simulink model "simple_streaming_txrx"  (Simulink 6.6)
settings: Solver=ode45  StartTime=0.0  StopTime=inf  RelTol=1e-3
InitFcn:
  | simple_streaming_init
StartFcn:
  | simple_streaming_init
undefined symbols (not defined in the file): dmf, gcbh, get, modConstellation_qam16, modConstellation_qam64, modConstellation_qpsk, rcosfir, symbolRomLen, txLSFR_initValues, txLSFR_polynomials, viqAvgLen, xlBlockLoadCallback, xlGetSimulinkPeriod
libraries: xbsIndex_r4 x506, commchan3 x2, commsink2 x1
(part 2 of 5)

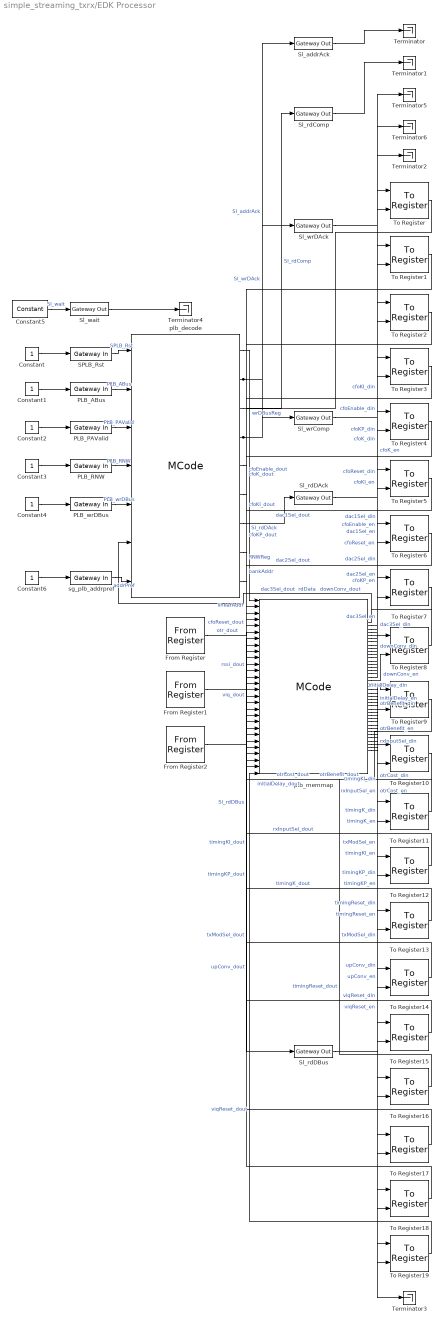
== system simple_streaming_txrx/EDK Processor ==
  Constant{,1..4,6} (6 alike) : Constant
  Constant5 : xbsIndex_r4/Constant  arith_type=Unsigned  const=0  n_bits=1  bin_pt=0  explicit_period=on  period=xlGetSimulinkPeriod(gcb)  equ=P=C  opselect=C  inp2=PCIN>>17  opr=+  inp1=P  carry=CIN  dbl_ovrd=off  block_type=constant
      settings: block_version=10.1.2
  From Register : xbsIndex_r4/From Register  shared_memory_name='otr'  init=0  period=xlGetSimulinkPeriod(gcb)  ownership=Owned and initialized elsewhere  arith_type=Unsigned  n_bits=32  bin_pt=0  dbl_ovrd=off  block_type=fromreg
      settings: AttributesFormatString=<< %<shared_memory_name> >>  infoedit="Register block that reads data to a shared memory register.  Delay of one sample period."  block_version=10.1.2
  From Register1 : xbsIndex_r4/From Register  shared_memory_name='rssi'  init=0  period=xlGetSimulinkPeriod(gcb)  ownership=Owned and initialized elsewhere  arith_type=Unsigned  n_bits=32  bin_pt=0  dbl_ovrd=off  block_type=fromreg
      settings: AttributesFormatString=<< %<shared_memory_name> >>  infoedit="Register block that reads data to a shared memory register.  Delay of one sample period."  block_version=10.1.2
  From Register2 : xbsIndex_r4/From Register  shared_memory_name='viq'  init=0  period=xlGetSimulinkPeriod(gcb)  ownership=Owned and initialized elsewhere  arith_type=Unsigned  n_bits=32  bin_pt=0  dbl_ovrd=off  block_type=fromreg
      settings: AttributesFormatString=<< %<shared_memory_name> >>  infoedit="Register block that reads data to a shared memory register.  Delay of one sample period."  block_version=10.1.2
  PLB_ABus : xbsIndex_r4/Gateway In  arith_type=Unsigned  n_bits=32  bin_pt=0  quantization="Round  (unbiased: +/- Inf)"  overflow=Saturate  period=xlGetSimulinkPeriod(gcb)  dbl_ovrd=off  timing_constraint=None  locs_specified=off  LOCs={}  block_type=gatewayin
      settings: infoedit="Gateway in block.  Converts inputs of type Simulink integer, double and fixed point to  Xilinx fixed point type.<P><P>Hardware notes:  In hardware these blocks become top level input ports."  sginterface={'Xilinx'=>{'jtaghwcosim'=>{'non_memory_mapped_port'=>'PLB_ABus'}},'iopad'=>{'constraint'=>'#'}}  block_version=10.1.2
  PLB_PAValid : xbsIndex_r4/Gateway In  arith_type=Unsigned  n_bits=1  bin_pt=0  quantization="Round  (unbiased: +/- Inf)"  overflow=Saturate  period=xlGetSimulinkPeriod(gcb)  dbl_ovrd=off  timing_constraint=None  locs_specified=off  LOCs={}  block_type=gatewayin
      settings: infoedit="Gateway in block.  Converts inputs of type Simulink integer, double and fixed point to  Xilinx fixed point type.<P><P>Hardware notes:  In hardware these blocks become top level input ports."  sginterface={'Xilinx'=>{'jtaghwcosim'=>{'non_memory_mapped_port'=>'PLB_PAValid'}},'iopad'=>{'constraint'=>'#'}}  block_version=10.1.2
  PLB_RNW : xbsIndex_r4/Gateway In  arith_type=Unsigned  n_bits=1  bin_pt=0  quantization="Round  (unbiased: +/- Inf)"  overflow=Saturate  period=xlGetSimulinkPeriod(gcb)  dbl_ovrd=off  timing_constraint=None  locs_specified=off  LOCs={}  block_type=gatewayin
      settings: infoedit="Gateway in block.  Converts inputs of type Simulink integer, double and fixed point to  Xilinx fixed point type.<P><P>Hardware notes:  In hardware these blocks become top level input ports."  sginterface={'Xilinx'=>{'jtaghwcosim'=>{'non_memory_mapped_port'=>'PLB_RNW'}},'iopad'=>{'constraint'=>'#'}}  block_version=10.1.2
  PLB_wrDBus : xbsIndex_r4/Gateway In  arith_type=Unsigned  n_bits=32  bin_pt=0  quantization="Round  (unbiased: +/- Inf)"  overflow=Saturate  period=xlGetSimulinkPeriod(gcb)  dbl_ovrd=off  timing_constraint=None  locs_specified=off  LOCs={}  block_type=gatewayin
      settings: infoedit="Gateway in block.  Converts inputs of type Simulink integer, double and fixed point to  Xilinx fixed point type.<P><P>Hardware notes:  In hardware these blocks become top level input ports."  sginterface={'Xilinx'=>{'jtaghwcosim'=>{'non_memory_mapped_port'=>'PLB_wrDBus'}},'iopad'=>{'constraint'=>'#'}}  block_version=10.1.2
  SPLB_Rst : xbsIndex_r4/Gateway In  arith_type=Unsigned  n_bits=1  bin_pt=0  quantization="Round  (unbiased: +/- Inf)"  overflow=Saturate  period=xlGetSimulinkPeriod(gcb)  dbl_ovrd=off  timing_constraint=None  locs_specified=off  LOCs={}  block_type=gatewayin
      settings: infoedit="Gateway in block.  Converts inputs of type Simulink integer, double and fixed point to  Xilinx fixed point type.<P><P>Hardware notes:  In hardware these blocks become top level input ports."  sginterface={'Xilinx'=>{'jtaghwcosim'=>{'non_memory_mapped_port'=>'SPLB_Rst'}},'iopad'=>{'constraint'=>'#'}}  block_version=10.1.2
  Sl_addrAck : xbsIndex_r4/Gateway Out  hdl_port=on  timing_constraint=None  locs_specified=off  LOCs={}  block_type=gatewayout
      settings: infoedit="Gateway out block.  Converts Xilinx fixed point inputs into ouputs of type Simulink integer, double, or fixed point.<P><P>Hardware notes:  In hardware these blocks become top level output ports or are discarded, depending on how they are configured."  sginterface={'Xilinx'=>{'jtaghwcosim'=>{'non_memory_mapped_port'=>'Sl_addrAck'}},'iopad'=>{'constraint'=>'#'}}  block_version=10.1.2
  Sl_rdComp : xbsIndex_r4/Gateway Out  hdl_port=on  timing_constraint=None  locs_specified=off  LOCs={}  block_type=gatewayout
      settings: infoedit="Gateway out block.  Converts Xilinx fixed point inputs into ouputs of type Simulink integer, double, or fixed point.<P><P>Hardware notes:  In hardware these blocks become top level output ports or are discarded, depending on how they are configured."  sginterface={'Xilinx'=>{'jtaghwcosim'=>{'non_memory_mapped_port'=>'Sl_rdComp'}},'iopad'=>{'constraint'=>'#'}}  block_version=10.1.2
  Sl_rdDAck : xbsIndex_r4/Gateway Out  hdl_port=on  timing_constraint=None  locs_specified=off  LOCs={}  block_type=gatewayout
      settings: infoedit="Gateway out block.  Converts Xilinx fixed point inputs into ouputs of type Simulink integer, double, or fixed point.<P><P>Hardware notes:  In hardware these blocks become top level output ports or are discarded, depending on how they are configured."  sginterface={'Xilinx'=>{'jtaghwcosim'=>{'non_memory_mapped_port'=>'Sl_rdDAck'}},'iopad'=>{'constraint'=>'#'}}  block_version=10.1.2
  Sl_rdDBus : xbsIndex_r4/Gateway Out  hdl_port=on  timing_constraint=None  locs_specified=off  LOCs={}  block_type=gatewayout
      settings: infoedit="Gateway out block.  Converts Xilinx fixed point inputs into ouputs of type Simulink integer, double, or fixed point.<P><P>Hardware notes:  In hardware these blocks become top level output ports or are discarded, depending on how they are configured."  sginterface={'Xilinx'=>{'jtaghwcosim'=>{'non_memory_mapped_port'=>'Sl_rdDBus'}},'iopad'=>{'constraint'=>'#'}}  block_version=10.1.2
  Sl_wait : xbsIndex_r4/Gateway Out  hdl_port=on  timing_constraint=None  locs_specified=off  LOCs={}  block_type=gatewayout
      settings: infoedit="Gateway out block.  Converts Xilinx fixed point inputs into ouputs of type Simulink integer, double, or fixed point.<P><P>Hardware notes:  In hardware these blocks become top level output ports or are discarded, depending on how they are configured."  sginterface={'Xilinx'=>{'jtaghwcosim'=>{'non_memory_mapped_port'=>'Sl_wait'}},'iopad'=>{'constraint'=>'#'}}  block_version=10.1.2
  Sl_wrComp : xbsIndex_r4/Gateway Out  hdl_port=on  timing_constraint=None  locs_specified=off  LOCs={}  block_type=gatewayout
      settings: infoedit="Gateway out block.  Converts Xilinx fixed point inputs into ouputs of type Simulink integer, double, or fixed point.<P><P>Hardware notes:  In hardware these blocks become top level output ports or are discarded, depending on how they are configured."  sginterface={'Xilinx'=>{'jtaghwcosim'=>{'non_memory_mapped_port'=>'Sl_wrComp'}},'iopad'=>{'constraint'=>'#'}}  block_version=10.1.2
  Sl_wrDAck : xbsIndex_r4/Gateway Out  hdl_port=on  timing_constraint=None  locs_specified=off  LOCs={}  block_type=gatewayout
      settings: infoedit="Gateway out block.  Converts Xilinx fixed point inputs into ouputs of type Simulink integer, double, or fixed point.<P><P>Hardware notes:  In hardware these blocks become top level output ports or are discarded, depending on how they are configured."  sginterface={'Xilinx'=>{'jtaghwcosim'=>{'non_memory_mapped_port'=>'Sl_wrDAck'}},'iopad'=>{'constraint'=>'#'}}  block_version=10.1.2
  Terminator{,1..6} (7 alike) : Terminator
  To Register : xbsIndex_r4/To Register  shared_memory_name='cfoEnable'  init=0  ownership=Owned and initialized elsewhere  explicit_data_type=on  arith_type=Unsigned  n_bits=1  bin_pt=0  dbl_ovrd=off  block_type=toreg
      settings: AttributesFormatString=<< %<shared_memory_name> >>  infoedit="Register block that writes data to a shared memory register.  Delay of one sample period."  block_version=10.1.2
  To Register1 : xbsIndex_r4/To Register  shared_memory_name='cfoK'  init=0  ownership=Owned and initialized elsewhere  explicit_data_type=on  arith_type=Unsigned  n_bits=32  bin_pt=0  dbl_ovrd=off  block_type=toreg
      settings: AttributesFormatString=<< %<shared_memory_name> >>  infoedit="Register block that writes data to a shared memory register.  Delay of one sample period."  block_version=10.1.2
  To Register10 : xbsIndex_r4/To Register  shared_memory_name='otrBenefit'  init=0  ownership=Owned and initialized elsewhere  explicit_data_type=on  arith_type=Unsigned  n_bits=32  bin_pt=0  dbl_ovrd=off  block_type=toreg
      settings: AttributesFormatString=<< %<shared_memory_name> >>  infoedit="Register block that writes data to a shared memory register.  Delay of one sample period."  block_version=10.1.2
  To Register11 : xbsIndex_r4/To Register  shared_memory_name='otrCost'  init=0  ownership=Owned and initialized elsewhere  explicit_data_type=on  arith_type=Unsigned  n_bits=32  bin_pt=0  dbl_ovrd=off  block_type=toreg
      settings: AttributesFormatString=<< %<shared_memory_name> >>  infoedit="Register block that writes data to a shared memory register.  Delay of one sample period."  block_version=10.1.2
  To Register12 : xbsIndex_r4/To Register  shared_memory_name='rxInputSel'  init=0  ownership=Owned and initialized elsewhere  explicit_data_type=on  arith_type=Unsigned  n_bits=2  bin_pt=0  dbl_ovrd=off  block_type=toreg
      settings: AttributesFormatString=<< %<shared_memory_name> >>  infoedit="Register block that writes data to a shared memory register.  Delay of one sample period."  block_version=10.1.2
  To Register13 : xbsIndex_r4/To Register  shared_memory_name='timingK'  init=0  ownership=Owned and initialized elsewhere  explicit_data_type=on  arith_type=Unsigned  n_bits=32  bin_pt=0  dbl_ovrd=off  block_type=toreg
      settings: AttributesFormatString=<< %<shared_memory_name> >>  infoedit="Register block that writes data to a shared memory register.  Delay of one sample period."  block_version=10.1.2
  To Register14 : xbsIndex_r4/To Register  shared_memory_name='timingKI'  init=0  ownership=Owned and initialized elsewhere  explicit_data_type=on  arith_type=Unsigned  n_bits=32  bin_pt=0  dbl_ovrd=off  block_type=toreg
      settings: AttributesFormatString=<< %<shared_memory_name> >>  infoedit="Register block that writes data to a shared memory register.  Delay of one sample period."  block_version=10.1.2
  To Register15 : xbsIndex_r4/To Register  shared_memory_name='timingKP'  init=0  ownership=Owned and initialized elsewhere  explicit_data_type=on  arith_type=Unsigned  n_bits=32  bin_pt=0  dbl_ovrd=off  block_type=toreg
      settings: AttributesFormatString=<< %<shared_memory_name> >>  infoedit="Register block that writes data to a shared memory register.  Delay of one sample period."  block_version=10.1.2
  To Register16 : xbsIndex_r4/To Register  shared_memory_name='timingReset'  init=0  ownership=Owned and initialized elsewhere  explicit_data_type=on  arith_type=Unsigned  n_bits=1  bin_pt=0  dbl_ovrd=off  block_type=toreg
      settings: AttributesFormatString=<< %<shared_memory_name> >>  infoedit="Register block that writes data to a shared memory register.  Delay of one sample period."  block_version=10.1.2
  To Register17 : xbsIndex_r4/To Register  shared_memory_name='txModSel'  init=0  ownership=Owned and initialized elsewhere  explicit_data_type=on  arith_type=Unsigned  n_bits=2  bin_pt=0  dbl_ovrd=off  block_type=toreg
      settings: AttributesFormatString=<< %<shared_memory_name> >>  infoedit="Register block that writes data to a shared memory register.  Delay of one sample period."  block_version=10.1.2
  To Register18 : xbsIndex_r4/To Register  shared_memory_name='upConv'  init=0  ownership=Owned and initialized elsewhere  explicit_data_type=on  arith_type=Unsigned  n_bits=32  bin_pt=0  dbl_ovrd=off  block_type=toreg
      settings: AttributesFormatString=<< %<shared_memory_name> >>  infoedit="Register block that writes data to a shared memory register.  Delay of one sample period."  block_version=10.1.2
  To Register19 : xbsIndex_r4/To Register  shared_memory_name='viqReset'  init=0  ownership=Owned and initialized elsewhere  explicit_data_type=on  arith_type=Unsigned  n_bits=1  bin_pt=0  dbl_ovrd=off  block_type=toreg
      settings: AttributesFormatString=<< %<shared_memory_name> >>  infoedit="Register block that writes data to a shared memory register.  Delay of one sample period."  block_version=10.1.2
  To Register2 : xbsIndex_r4/To Register  shared_memory_name='cfoKI'  init=0  ownership=Owned and initialized elsewhere  explicit_data_type=on  arith_type=Unsigned  n_bits=32  bin_pt=0  dbl_ovrd=off  block_type=toreg
      settings: AttributesFormatString=<< %<shared_memory_name> >>  infoedit="Register block that writes data to a shared memory register.  Delay of one sample period."  block_version=10.1.2
  To Register3 : xbsIndex_r4/To Register  shared_memory_name='cfoKP'  init=0  ownership=Owned and initialized elsewhere  explicit_data_type=on  arith_type=Unsigned  n_bits=32  bin_pt=0  dbl_ovrd=off  block_type=toreg
      settings: AttributesFormatString=<< %<shared_memory_name> >>  infoedit="Register block that writes data to a shared memory register.  Delay of one sample period."  block_version=10.1.2
  To Register4 : xbsIndex_r4/To Register  shared_memory_name='cfoReset'  init=0  ownership=Owned and initialized elsewhere  explicit_data_type=on  arith_type=Unsigned  n_bits=1  bin_pt=0  dbl_ovrd=off  block_type=toreg
      settings: AttributesFormatString=<< %<shared_memory_name> >>  infoedit="Register block that writes data to a shared memory register.  Delay of one sample period."  block_version=10.1.2
  To Register5 : xbsIndex_r4/To Register  shared_memory_name='dac1Sel'  init=0  ownership=Owned and initialized elsewhere  explicit_data_type=on  arith_type=Unsigned  n_bits=2  bin_pt=0  dbl_ovrd=off  block_type=toreg
      settings: AttributesFormatString=<< %<shared_memory_name> >>  infoedit="Register block that writes data to a shared memory register.  Delay of one sample period."  block_version=10.1.2
  To Register6 : xbsIndex_r4/To Register  shared_memory_name='dac2Sel'  init=0  ownership=Owned and initialized elsewhere  explicit_data_type=on  arith_type=Unsigned  n_bits=2  bin_pt=0  dbl_ovrd=off  block_type=toreg
      settings: AttributesFormatString=<< %<shared_memory_name> >>  infoedit="Register block that writes data to a shared memory register.  Delay of one sample period."  block_version=10.1.2
  To Register7 : xbsIndex_r4/To Register  shared_memory_name='dac3Sel'  init=0  ownership=Owned and initialized elsewhere  explicit_data_type=on  arith_type=Unsigned  n_bits=1  bin_pt=0  dbl_ovrd=off  block_type=toreg
      settings: AttributesFormatString=<< %<shared_memory_name> >>  infoedit="Register block that writes data to a shared memory register.  Delay of one sample period."  block_version=10.1.2
  To Register8 : xbsIndex_r4/To Register  shared_memory_name='downConv'  init=0  ownership=Owned and initialized elsewhere  explicit_data_type=on  arith_type=Unsigned  n_bits=32  bin_pt=0  dbl_ovrd=off  block_type=toreg
      settings: AttributesFormatString=<< %<shared_memory_name> >>  infoedit="Register block that writes data to a shared memory register.  Delay of one sample period."  block_version=10.1.2
  To Register9 : xbsIndex_r4/To Register  shared_memory_name='initialDelay'  init=0  ownership=Owned and initialized elsewhere  explicit_data_type=on  arith_type=Unsigned  n_bits=2  bin_pt=0  dbl_ovrd=off  block_type=toreg
      settings: AttributesFormatString=<< %<shared_memory_name> >>  infoedit="Register block that writes data to a shared memory register.  Delay of one sample period."  block_version=10.1.2
  plb_decode : xbsIndex_r4/MCode  mfname=xlmax  explicit_period=off  period=1  dbl_ovrd=off  enable_stdout=off  enable_debug=off  mfilecontent=|  suppress_output=1  defparams={}  hide_port_list={}  block_type=mcode
      | function [wrDBusReg, addrAck, rdComp, wrDAck, bankAddr, RNWReg, rdDAck, rdDBus, linearAddr] = ...
      |     plb_bus_decode(plbRst, plbABus, plbPAValid, plbRNW, plbWrDBus, rdData, addrPref)
      | 
      | % constant variables (TODO: should pass from outside)
      | ADDRPREF_LEN = 20;
      | BANKADDR_LEN = 2;
      | LINEARADDR_LEN = 8;
      | ABUS_LEN = 32;
      | DBUS_LEN = 32;
      | 
      | % declare and initialize persistent variables
      | % register input bus signals
      | persistent plbRstReg_, plbRstReg_ = xl_state(0, {xlBoolean});
      | persistent plbABusReg_, plbABusReg_ = xl_state(0, {xlUnsigned, ABUS_LEN, 0});
      | persistent plbPAValidReg_, plbPAValidReg_ = xl_state(0, {xlBoolean});
      | persistent plbRNWReg_, plbRNWReg_ = xl_state(0, {xlUnsigned, 1, 0});
      | persistent plbWrDBusReg_, plbWrDBusReg_ = xl_state(0, {xlUnsigned, DBUS_LEN, 0});
      | 
      | % ===== rest of the outputs =====
      | 
      | bankAddr   = xl_slice(plbABusReg_, 2+BANKADDR_LEN+LINEARADDR_LEN-1, 2+LINEARADDR_LEN);
      | linearAddr = xl_slice(plbABusReg_, 2+LINEARADDR_LEN-1, 2);
      | RNWReg = plbRNWReg_;
      | wrDBusReg = plbWrDBusReg_;
      | 
      | % ===== p_select =====
      | 
      | % register PAValid
      | persistent aValidReg, aValidReg = xl_state(0, {xlBoolean});
      | aValidReg = plbPAValidReg_;
      | 
      | % extract and register the address prefix
      | addrPref_in = xl_slice(plbABusReg_, xl_nbits(plbABusReg_)-1, xl_nbits(plbABusReg_)-ADDRPREF_LEN);
      | if addrPref_in == addrPref
      |     ps1 = true;
      | else 
      |     ps1 = false;
      | end 
      | 
      | persistent ps1Reg, ps1Reg = xl_state(0, ps1);
      | ps1Reg = ps1;
      | 
      | ps = xl_and(ps1Reg, aValidReg);
      | 
      | % ===== addrAck =====
      | 
      | % register ps
      | persistent psReg, psReg = xl_state(0, ps);
      | 
      | addrAck = xfix({xlUnsigned, 1, 0}, xl_and(xl_not(plbRstReg_), ps, xl_not(psReg)));
      | 
      | psReg = ps;
      | 
      | % ===== rdComp, rd/wr DAck =====
      |  
      | rdComp1 = xfix({xlUnsigned, 1, 0}, xl_and(addrAck, RNWReg));
      | 
      | NUM_rdCompDelay = 3;
      | persistent rdCompDelay, rdCompDelay = xl_state(zeros(1, NUM_rdCompDelay), rdComp1, NUM_rdCompDelay);
      | rdComp2 = rdCompDelay.back;
      | rdCompDelay.push_front_pop_back(rdComp1);
      | 
      | persistent rdCompReg, rdCompReg = xl_state(0, rdComp1);
      | rdComp = rdCompReg;
      | rdCompReg = rdComp2;
      | 
      | persistent rdDAckReg, rdDAckReg = xl_state(0, rdComp1);
      | rdDAck = rdDAckReg;
      | rdDAckReg = rdComp;
      | 
      | persistent wrDAckReg, wrDAckReg = xl_state(0, addrAck);
      | wrDAck = wrDAckReg;
      | wrDAckReg = xl_and(addrAck, xl_not(RNWReg));
      | 
      | % ===== rdDBus =====
      | 
      | rdSel = xl_or(rdComp2, rdComp);
      | 
      | if rdSel == 1
      |     rdDBus1 = rdData;
      | else
      |     rdDBus1 = 0;
      | end % if
      | 
      | persistent rdDBusReg, rdDBusReg = xl_state(0, rdDBus1);
      | rdDBus = rdDBusReg;
      | rdDBusReg = rdDBus1;
      | 
      | % rdDBus = xl_concat(rdDBus32, rdDBus32);
      | % rdDBus = rdDBus32;
      | 
      | % ===== update the persistent variables =====
      | 
      | plbRstReg_ = plbRst;
      | plbABusReg_ = plbABus;
      | plbPAValidReg_ = plbPAValid;
      | plbRNWReg_ = plbRNW;
      | plbWrDBusReg_ = xl_slice(plbWrDBus, DBUS_LEN-1, 0);
      settings: block_version=10.1.2
  plb_memmap : xbsIndex_r4/MCode  mfname=xlmax  explicit_period=off  period=1  dbl_ovrd=off  enable_stdout=off  enable_debug=off  mfilecontent=|  suppress_output=1  defparams={}  hide_port_list={}  block_type=mcode
      | function [read_bank_out, sm_cfoEnable_din, sm_cfoEnable_en, sm_cfoK_din, sm_cfoK_en, sm_cfoKI_din, sm_cfoKI_en, sm_cfoKP_din, sm_cfoKP_en, sm_cfoReset_din, sm_cfoReset_en, sm_dac1Sel_din, sm_dac1Sel_en, sm_dac2Sel_din, sm_dac2Sel_en, sm_dac3Sel_din, sm_dac3Sel_en, sm_downConv_din, sm_downConv_en, sm_initialDelay_din, sm_initialDelay_en, sm_otrBenefit_din, sm_otrBenefit_en, sm_otrCost_din, sm_otrCost_en, sm_rxInputSel_din, sm_rxInputSel_en, sm_timingK_din, sm_timingK_en, sm_timingKI_din, sm_timingKI_en, sm_timingKP_din, sm_timingKP_en, sm_timingReset_din, sm_timingReset_en, sm_txModSel_din, sm_txModSel_en, sm_upConv_din, sm_upConv_en, sm_viqReset_din, sm_viqReset_en] = plb_memmap_select(wrDBus, bankAddr, linearAddr, RNWReg, addrAck, sm_otr, sm_rssi, sm_viq, sm_cfoEnable, sm_cfoK, sm_cfoKI, sm_cfoKP, sm_cfoReset, sm_dac1Sel, sm_dac2Sel, sm_dac3Sel, sm_downConv, sm_initialDelay, sm_otrBenefit, sm_otrCost, sm_rxInputSel, sm_timingK, sm_timingKI, sm_timingKP, sm_timingReset, sm_txModSel, sm_upConv, sm_viqReset)
      | 
      | 
      | % connvert the input data to UFix_32_0 (the bus data type)
      | % 'From Register' blocks
      | % sm_otr_bus = xfix({xlUnsigned, 32, 0}, 0);
      | sm_otr_bus = xl_force(sm_otr, xlUnsigned, 0);
      | 
      | % sm_rssi_bus = xfix({xlUnsigned, 32, 0}, 0);
      | sm_rssi_bus = xl_force(sm_rssi, xlUnsigned, 0);
      | 
      | % sm_viq_bus = xfix({xlUnsigned, 32, 0}, 0);
      | sm_viq_bus = xl_force(sm_viq, xlUnsigned, 0);
      | 
      | % 'To Register' blocks
      | % sm_cfoEnable_dout = xfix({xlUnsigned, 32, 0}, 0);
      | sm_cfoEnable_dout = xl_force(sm_cfoEnable, xlUnsigned, 0);
      | 
      | % sm_cfoK_dout = xfix({xlUnsigned, 32, 0}, 0);
      | sm_cfoK_dout = xl_force(sm_cfoK, xlUnsigned, 0);
      | 
      | % sm_cfoKI_dout = xfix({xlUnsigned, 32, 0}, 0);
      | sm_cfoKI_dout = xl_force(sm_cfoKI, xlUnsigned, 0);
      | 
      | % sm_cfoKP_dout = xfix({xlUnsigned, 32, 0}, 0);
      | sm_cfoKP_dout = xl_force(sm_cfoKP, xlUnsigned, 0);
      | 
      | % sm_cfoReset_dout = xfix({xlUnsigned, 32, 0}, 0);
      | sm_cfoReset_dout = xl_force(sm_cfoReset, xlUnsigned, 0);
      | 
      | % sm_dac1Sel_dout = xfix({xlUnsigned, 32, 0}, 0);
      | sm_dac1Sel_dout = xl_force(sm_dac1Sel, xlUnsigned, 0);
      | 
      | % sm_dac2Sel_dout = xfix({xlUnsigned, 32, 0}, 0);
      | sm_dac2Sel_dout = xl_force(sm_dac2Sel, xlUnsigned, 0);
      | 
      | % sm_dac3Sel_dout = xfix({xlUnsigned, 32, 0}, 0);
      | sm_dac3Sel_dout = xl_force(sm_dac3Sel, xlUnsigned, 0);
      | 
      | % sm_downConv_dout = xfix({xlUnsigned, 32, 0}, 0);
      | sm_downConv_dout = xl_force(sm_downConv, xlUnsigned, 0);
      | 
      | % sm_initialDelay_dout = xfix({xlUnsigned, 32, 0}, 0);
      | sm_initialDelay_dout = xl_force(sm_initialDelay, xlUnsigned, 0);
      | 
      | % sm_otrBenefit_dout = xfix({xlUnsigned, 32, 0}, 0);
      | sm_otrBenefit_dout = xl_force(sm_otrBenefit, xlUnsigned, 0);
      | 
      | % sm_otrCost_dout = xfix({xlUnsigned, 32, 0}, 0);
      | sm_otrCost_dout = xl_force(sm_otrCost, xlUnsigned, 0);
      | 
      | % sm_rxInputSel_dout = xfix({xlUnsigned, 32, 0}, 0);
      | sm_rxInputSel_dout = xl_force(sm_rxInputSel, xlUnsigned, 0);
      | 
      | % sm_timingK_dout = xfix({xlUnsigned, 32, 0}, 0);
      | sm_timingK_dout = xl_force(sm_timingK, xlUnsigned, 0);
      | 
      | % sm_timingKI_dout = xfix({xlUnsigned, 32, 0}, 0);
      | sm_timingKI_dout = xl_force(sm_timingKI, xlUnsigned, 0);
      | 
      | % sm_timingKP_dout = xfix({xlUnsigned, 32, 0}, 0);
      | sm_timingKP_dout = xl_force(sm_timingKP, xlUnsigned, 0);
      | 
      | % sm_timingReset_dout = xfix({xlUnsigned, 32, 0}, 0);
      | sm_timingReset_dout = xl_force(sm_timingReset, xlUnsigned, 0);
      | 
      | % sm_txModSel_dout = xfix({xlUnsigned, 32, 0}, 0);
      | sm_txModSel_dout = xl_force(sm_txModSel, xlUnsigned, 0);
      | 
      | % sm_upConv_dout = xfix({xlUnsigned, 32, 0}, 0);
      | sm_upConv_dout = xl_force(sm_upConv, xlUnsigned, 0);
      | 
      | % sm_viqReset_dout = xfix({xlUnsigned, 32, 0}, 0);
      | sm_viqReset_dout = xl_force(sm_viqReset, xlUnsigned, 0);
      | 
      | % 'From FIFO' blocks
      | % 'To FIFO' blocks
      | % 'Shared Memory' blocks
      | 
      | % 'dout' ports of 'From Register' blocks
      | 
      | % registered register mux output
      | persistent reg_bank_out_reg; reg_bank_out_reg = xl_state(0, {xlUnsigned, 32, 0});
      | reg_bank_out = reg_bank_out_reg;
      | 
      | if linearAddr == 20
      |     reg_bank_out_reg = sm_otr_bus;
      | elseif linearAddr == 21
      |     reg_bank_out_reg = sm_rssi_bus;
      | elseif linearAddr == 22
      |     reg_bank_out_reg = sm_viq_bus;
      | elseif linearAddr == 0
      |     reg_bank_out_reg = sm_cfoEnable_dout;
      | elseif linearAddr == 1
      |     reg_bank_out_reg = sm_cfoK_dout;
      | elseif linearAddr == 2
      |     reg_bank_out_reg = sm_cfoKI_dout;
      | elseif linearAddr == 3
      |     reg_bank_out_reg = sm_cfoKP_dout;
      | elseif linearAddr == 4
      |     reg_bank_out_reg = sm_cfoReset_dout;
      | elseif linearAddr == 5
      |     reg_bank_out_reg = sm_dac1Sel_dout;
      | elseif linearAddr == 6
      |     reg_bank_out_reg = sm_dac2Sel_dout;
      | elseif linearAddr == 7
      |     reg_bank_out_reg = sm_dac3Sel_dout;
      | elseif linearAddr == 8
      |     reg_bank_out_reg = sm_downConv_dout;
      | elseif linearAddr == 9
      |     reg_bank_out_reg = sm_initialDelay_dout;
      | elseif linearAddr == 10
      |     reg_bank_out_reg = sm_otrBenefit_dout;
      | elseif linearAddr == 11
      |     reg_bank_out_reg = sm_otrCost_dout;
      | elseif linearAddr == 12
      |     reg_bank_out_reg = sm_rxInputSel_dout;
      | elseif linearAddr == 13
      |     reg_bank_out_reg = sm_timingK_dout;
      | elseif linearAddr == 14
      |     reg_bank_out_reg = sm_timingKI_dout;
      | elseif linearAddr == 15
      |     reg_bank_out_reg = sm_timingKP_dout;
      | elseif linearAddr == 16
      |     reg_bank_out_reg = sm_timingReset_dout;
      | elseif linearAddr == 17
      |     reg_bank_out_reg = sm_txModSel_dout;
      | elseif linearAddr == 18
      |     reg_bank_out_reg = sm_upConv_dout;
      | elseif linearAddr == 19
      |     reg_bank_out_reg = sm_viqReset_dout;
      | end
      | 
      | 
      | % 'From FIFO' and 'To FIFO' blocks
      | 
      | 
      | 
      | 
      | 
      | opCode = xl_concat(addrAck, RNWReg, bankAddr, linearAddr);
      | 
      | % 'Shared Memory' blocks
      | 
      | 
      | 
      | 
      | 
      | % 'din' ports of 'Shared Memory' blocks
      | 
      | 
      | % 'we' ports of 'Shared Memory' blocks
      | 
      | 
      | % 'addr' ports of 'Shared Memory' blocks
      | 
      | 
      | % 're' ports of 'From FIFO' blocks
      | 
      | 
      | % 'en' ports of 'To Register' blocks
      | if opCode == xl_concat(xfix({xlUnsigned, 4, 0}, 10), ...
      |                        xfix({xlUnsigned, xl_nbits(linearAddr), 0}, 0))
      |     sm_cfoEnable_en = true;
      | else
      |     sm_cfoEnable_en = false;
      | end
      | if opCode == xl_concat(xfix({xlUnsigned, 4, 0}, 10), ...
      |                        xfix({xlUnsigned, xl_nbits(linearAddr), 0}, 1))
      |     sm_cfoK_en = true;
      | else
      |     sm_cfoK_en = false;
      | end
      | if opCode == xl_concat(xfix({xlUnsigned, 4, 0}, 10), ...
      |                        xfix({xlUnsigned, xl_nbits(linearAddr), 0}, 2))
      |     sm_cfoKI_en = true;
      | else
      |     sm_cfoKI_en = false;
      | end
      | if opCode == xl_concat(xfix({xlUnsigned, 4, 0}, 10), ...
      |                        xfix({xlUnsigned, xl_nbits(linearAddr), 0}, 3))
      |     sm_cfoKP_en = true;
      | else
      |     sm_cfoKP_en = false;
      | end
      | if opCode == xl_concat(xfix({xlUnsigned, 4, 0}, 10), ...
      |                        xfix({xlUnsigned, xl_nbits(linearAddr), 0}, 4))
      |     sm_cfoReset_en = true;
      | else
      |     sm_cfoReset_en = false;
      | end
      | if opCode == xl_concat(xfix({xlUnsigned, 4, 0}, 10), ...
      |                        xfix({xlUnsigned, xl_nbits(linearAddr), 0}, 5))
      |     sm_dac1Sel_en = true;
      | else
      |     sm_dac1Sel_en = false;
      | end
      | if opCode == xl_concat(xfix({xlUnsigned, 4, 0}, 10), ...
      |                        xfix({xlUnsigned, xl_nbits(linearAddr), 0}, 6))
      |     sm_dac2Sel_en = true;
      | else
      |     sm_dac2Sel_en = false;
      | end
      | if opCode == xl_concat(xfix({xlUnsigned, 4, 0}, 10), ...
      |                        xfix({xlUnsigned, xl_nbits(linearAddr), 0}, 7))
      |     sm_dac3Sel_en = true;
      | else
      |     sm_dac3Sel_en = false;
      | end
      | if opCode == xl_concat(xfix({xlUnsigned, 4, 0}, 10), ...
      |                        xfix({xlUnsigned, xl_nbits(linearAddr), 0}, 8))
      |     sm_downConv_en = true;
      | else
      |     sm_downConv_en = false;
      | end
      | if opCode == xl_concat(xfix({xlUnsigned, 4, 0}, 10), ...
      |                        xfix({xlUnsigned, xl_nbits(linearAddr), 0}, 9))
      |     sm_initialDelay_en = true;
      | else
      |     sm_initialDelay_en = false;
      | end
      | if opCode == xl_concat(xfix({xlUnsigned, 4, 0}, 10), ...
      |                        xfix({xlUnsigned, xl_nbits(linearAddr), 0}, 10))
      |     sm_otrBenefit_en = true;
      | else
      |     sm_otrBenefit_en = false;
      | end
      | if opCode == xl_concat(xfix({xlUnsigned, 4, 0}, 10), ...
      |                        xfix({xlUnsigned, xl_nbits(linearAddr), 0}, 11))
      |     sm_otrCost_en = true;
      | else
      |     sm_otrCost_en = false;
      | end
      | if opCode == xl_concat(xfix({xlUnsigned, 4, 0}, 10), ...
      |                        xfix({xlUnsigned, xl_nbits(linearAddr), 0}, 12))
      |     sm_rxInputSel_en = true;
      | else
      |     sm_rxInputSel_en = false;
      | end
      | if opCode == xl_concat(xfix({xlUnsigned, 4, 0}, 10), ...
      |                        xfix({xlUnsigned, xl_nbits(linearAddr), 0}, 13))
      |     sm_timingK_en = true;
      | else
      |     sm_timingK_en = false;
      | end
      | if opCode == xl_concat(xfix({xlUnsigned, 4, 0}, 10), ...
      |                        xfix({xlUnsigned, xl_nbits(linearAddr), 0}, 14))
      |     sm_timingKI_en = true;
      | else
      |     sm_timingKI_en = false;
      | end
      | if opCode == xl_concat(xfix({xlUnsigned, 4, 0}, 10), ...
      |                        xfix({xlUnsigned, xl_nbits(linearAddr), 0}, 15))
      |     sm_timingKP_en = true;
      | else
      |     sm_timingKP_en = false;
      | end
      | if opCode == xl_concat(xfix({xlUnsigned, 4, 0}, 10), ...
      |                        xfix({xlUnsigned, xl_nbits(linearAddr), 0}, 16))
      |     sm_timingReset_en = true;
      | else
      |     sm_timingReset_en = false;
      | end
      | if opCode == xl_concat(xfix({xlUnsigned, 4, 0}, 10), ...
      |                        xfix({xlUnsigned, xl_nbits(linearAddr), 0}, 17))
      |     sm_txModSel_en = true;
      | else
      |     sm_txModSel_en = false;
      | end
      | if opCode == xl_concat(xfix({xlUnsigned, 4, 0}, 10), ...
      |                        xfix({xlUnsigned, xl_nbits(linearAddr), 0}, 18))
      |     sm_upConv_en = true;
      | else
      |     sm_upConv_en = false;
      | end
      | if opCode == xl_concat(xfix({xlUnsigned, 4, 0}, 10), ...
      |                        xfix({xlUnsigned, xl_nbits(linearAddr), 0}, 19))
      |     sm_viqReset_en = true;
      | else
      |     sm_viqReset_en = false;
      | end
      | 
      | 
      | % 'din' ports of 'To FIFO' blocks
      | 
      | 
      | % 'we' ports of 'To FIFO' blocks
      | 
      | 
      | % 'din' ports of 'To Register' blocks
      | sm_cfoEnable_din = xl_force(xl_slice(wrDBus, 1 - 1, 0), ...
      |                                  xlUnsigned, ...
      |                                  0);
      | sm_cfoK_din = xl_force(xl_slice(wrDBus, 32 - 1, 0), ...
      |                                  xlUnsigned, ...
      |                                  0);
      | sm_cfoKI_din = xl_force(xl_slice(wrDBus, 32 - 1, 0), ...
      |                                  xlUnsigned, ...
      |                                  0);
      | sm_cfoKP_din = xl_force(xl_slice(wrDBus, 32 - 1, 0), ...
      |                                  xlUnsigned, ...
      |                                  0);
      | sm_cfoReset_din = xl_force(xl_slice(wrDBus, 1 - 1, 0), ...
      |                                  xlUnsigned, ...
      |                                  0);
      | sm_dac1Sel_din = xl_force(xl_slice(wrDBus, 2 - 1, 0), ...
      |                                  xlUnsigned, ...
      |                                  0);
      | sm_dac2Sel_din = xl_force(xl_slice(wrDBus, 2 - 1, 0), ...
      |                                  xlUnsigned, ...
      |                                  0);
      | sm_dac3Sel_din = xl_force(xl_slice(wrDBus, 1 - 1, 0), ...
      |                                  xlUnsigned, ...
      |                                  0);
      | sm_downConv_din = xl_force(xl_slice(wrDBus, 32 - 1, 0), ...
      |                                  xlUnsigned, ...
      |                                  0);
      | sm_initialDelay_din = xl_force(xl_slice(wrDBus, 2 - 1, 0), ...
      |                                  xlUnsigned, ...
      |                                  0);
      | sm_otrBenefit_din = xl_force(xl_slice(wrDBus, 32 - 1, 0), ...
      |                                  xlUnsigned, ...
      |                                  0);
      | sm_otrCost_din = xl_force(xl_slice(wrDBus, 32 - 1, 0), ...
      |                                  xlUnsigned, ...
      |                                  0);
      | sm_rxInputSel_din = xl_force(xl_slice(wrDBus, 2 - 1, 0), ...
      |                                  xlUnsigned, ...
      |                                  0);
      | sm_timingK_din = xl_force(xl_slice(wrDBus, 32 - 1, 0), ...
      |                                  xlUnsigned, ...
      |                                  0);
      | sm_timingKI_din = xl_force(xl_slice(wrDBus, 32 - 1, 0), ...
      |                                  xlUnsigned, ...
      |                                  0);
      | sm_timingKP_din = xl_force(xl_slice(wrDBus, 32 - 1, 0), ...
      |                                  xlUnsigned, ...
      |                                  0);
      | sm_timingReset_din = xl_force(xl_slice(wrDBus, 1 - 1, 0), ...
      |                                  xlUnsigned, ...
      |                                  0);
      | sm_txModSel_din = xl_force(xl_slice(wrDBus, 2 - 1, 0), ...
      |                                  xlUnsigned, ...
      |                                  0);
      | sm_upConv_din = xl_force(xl_slice(wrDBus, 32 - 1, 0), ...
      |                                  xlUnsigned, ...
      |                                  0);
      | sm_viqReset_din = xl_force(xl_slice(wrDBus, 1 - 1, 0), ...
      |                                  xlUnsigned, ...
      |                                  0);
      | 
      | 
      | persistent read_bank_out_reg; read_bank_out_reg = xl_state(0, {xlUnsigned, 32, 0});
      | read_bank_out = read_bank_out_reg;
      | 
      | persistent bankAddr_reg; bankAddr_reg = xl_state(0, bankAddr);
      | 
      | if bankAddr_reg == 0
      |     % Bank 0: Shared Memories
      |     read_bank_out_reg = 0;
      | elseif bankAddr_reg == 1
      |     % Bank 1: From/To FIFOs
      |     read_bank_out_reg =  0;
      | elseif bankAddr_reg == 2
      |     % Bank 1: From/To Registers
      |     read_bank_out_reg = reg_bank_out;
      | elseif bankAddr_reg == 3
      |     % Bank 1: Configure Registers
      |     read_bank_out_reg = 0;
      | end
      | 
      | bankAddr_reg = bankAddr;
      settings: block_version=10.1.2
  sg_plb_addrpref : xbsIndex_r4/Gateway In  arith_type=Unsigned  n_bits=20  bin_pt=0  quantization="Round  (unbiased: +/- Inf)"  overflow=Saturate  period=xlGetSimulinkPeriod(gcb)  dbl_ovrd=off  timing_constraint=None  locs_specified=off  LOCs={}  block_type=gatewayin
      settings: infoedit="Gateway in block.  Converts inputs of type Simulink integer, double and fixed point to  Xilinx fixed point type.<P><P>Hardware notes:  In hardware these blocks become top level input ports."  sginterface={'Xilinx'=>{'jtaghwcosim'=>{'non_memory_mapped_port'=>'sg_plb_addrpref'}},'iopad'=>{'constraint'=>'#'}}  block_version=10.1.2
  wires:
  plb_decode/2 -> plb_memmap/5, Sl_addrAck/1  "Sl_addrAck"
  plb_decode/4 -> Sl_wrDAck/1, Sl_wrComp/1  "Sl_wrDAck"
  plb_memmap/41 -> To Register19/2  "viqReset_en"
  plb_memmap/40 -> To Register19/1  "viqReset_din"
  plb_memmap/39 -> To Register18/2  "upConv_en"
  plb_memmap/38 -> To Register18/1  "upConv_din"
  plb_memmap/37 -> To Register17/2  "txModSel_en"
  plb_memmap/36 -> To Register17/1  "txModSel_din"
  plb_memmap/35 -> To Register16/2  "timingReset_en"
  plb_memmap/34 -> To Register16/1  "timingReset_din"
  plb_memmap/33 -> To Register15/2  "timingKP_en"
  plb_memmap/32 -> To Register15/1  "timingKP_din"
  plb_memmap/31 -> To Register14/2  "timingKI_en"
  plb_memmap/30 -> To Register14/1  "timingKI_din"
  plb_memmap/29 -> To Register13/2  "timingK_en"
  plb_memmap/28 -> To Register13/1  "timingK_din"
  plb_memmap/27 -> To Register12/2  "rxInputSel_en"
  plb_memmap/26 -> To Register12/1  "rxInputSel_din"
  plb_memmap/25 -> To Register11/2  "otrCost_en"
  plb_memmap/24 -> To Register11/1  "otrCost_din"
  plb_memmap/23 -> To Register10/2  "otrBenefit_en"
  plb_memmap/22 -> To Register10/1  "otrBenefit_din"
  plb_memmap/21 -> To Register9/2  "initialDelay_en"
  plb_memmap/20 -> To Register9/1  "initialDelay_din"
  plb_memmap/19 -> To Register8/2  "downConv_en"
  plb_memmap/18 -> To Register8/1  "downConv_din"
  plb_memmap/17 -> To Register7/2  "dac3Sel_en"
  plb_memmap/16 -> To Register7/1  "dac3Sel_din"
  plb_memmap/15 -> To Register6/2  "dac2Sel_en"
  plb_memmap/14 -> To Register6/1  "dac2Sel_din"
  plb_memmap/13 -> To Register5/2  "dac1Sel_en"
  plb_memmap/12 -> To Register5/1  "dac1Sel_din"
  plb_memmap/11 -> To Register4/2  "cfoReset_en"
  plb_memmap/10 -> To Register4/1  "cfoReset_din"
  plb_memmap/9 -> To Register3/2  "cfoKP_en"
  plb_memmap/8 -> To Register3/1  "cfoKP_din"
  plb_memmap/7 -> To Register2/2  "cfoKI_en"
  plb_memmap/6 -> To Register2/1  "cfoKI_din"
  plb_memmap/5 -> To Register1/2  "cfoK_en"
  plb_memmap/4 -> To Register1/1  "cfoK_din"
  plb_memmap/3 -> To Register/2  "cfoEnable_en"
  plb_memmap/2 -> To Register/1  "cfoEnable_din"
  plb_memmap/1 -> plb_decode/6  "rdData"
  To Register19/1 -> plb_memmap/28  "viqReset_dout"
  To Register18/1 -> plb_memmap/27  "upConv_dout"
  To Register17/1 -> plb_memmap/26  "txModSel_dout"
  To Register16/1 -> plb_memmap/25  "timingReset_dout"
  To Register15/1 -> plb_memmap/24  "timingKP_dout"
  To Register14/1 -> plb_memmap/23  "timingKI_dout"
  To Register13/1 -> plb_memmap/22  "timingK_dout"
  To Register12/1 -> plb_memmap/21  "rxInputSel_dout"
  To Register11/1 -> plb_memmap/20  "otrCost_dout"
  To Register10/1 -> plb_memmap/19  "otrBenefit_dout"
  To Register9/1 -> plb_memmap/18  "initialDelay_dout"
  To Register8/1 -> plb_memmap/17  "downConv_dout"
  To Register7/1 -> plb_memmap/16  "dac3Sel_dout"
  To Register6/1 -> plb_memmap/15  "dac2Sel_dout"
  To Register5/1 -> plb_memmap/14  "dac1Sel_dout"
  To Register4/1 -> plb_memmap/13  "cfoReset_dout"
  To Register3/1 -> plb_memmap/12  "cfoKP_dout"
  To Register2/1 -> plb_memmap/11  "cfoKI_dout"
  To Register1/1 -> plb_memmap/10  "cfoK_dout"
  To Register/1 -> plb_memmap/9  "cfoEnable_dout"
  From Register2/1 -> plb_memmap/8  "viq_dout"
  From Register1/1 -> plb_memmap/7  "rssi_dout"
  From Register/1 -> plb_memmap/6  "otr_dout"
  plb_decode/6 -> plb_memmap/4  "RNWReg"
  plb_decode/9 -> plb_memmap/3  "linearAddr"
  plb_decode/5 -> plb_memmap/2  "bankAddr"
  plb_decode/1 -> plb_memmap/1  "wrDBusReg"
  plb_decode/8 -> Sl_rdDBus/1  "Sl_rdDBus"
  plb_decode/7 -> Sl_rdDAck/1  "Sl_rdDAck"
  plb_decode/3 -> Sl_rdComp/1  "Sl_rdComp"
  sg_plb_addrpref/1 -> plb_decode/7  "addrPref"
  PLB_wrDBus/1 -> plb_decode/5  "PLB_wrDBus"
  PLB_RNW/1 -> plb_decode/4  "PLB_RNW"
  PLB_PAValid/1 -> plb_decode/3  "PLB_PAValid"
  PLB_ABus/1 -> plb_decode/2  "PLB_ABus"
  SPLB_Rst/1 -> plb_decode/1  "SPLB_Rst"
  Constant6/1 -> sg_plb_addrpref/1
  Constant5/1 -> Sl_wait/1  "Sl_wait"
  Constant4/1 -> PLB_wrDBus/1
  Constant3/1 -> PLB_RNW/1
  Constant2/1 -> PLB_PAValid/1
  Constant1/1 -> PLB_ABus/1
  Constant/1 -> SPLB_Rst/1
  Sl_wrComp/1 -> Terminator6/1
  Sl_wrDAck/1 -> Terminator5/1
  Sl_wait/1 -> Terminator4/1
  Sl_rdDBus/1 -> Terminator3/1
  Sl_rdDAck/1 -> Terminator2/1
  Sl_rdComp/1 -> Terminator1/1
  Sl_addrAck/1 -> Terminator/1

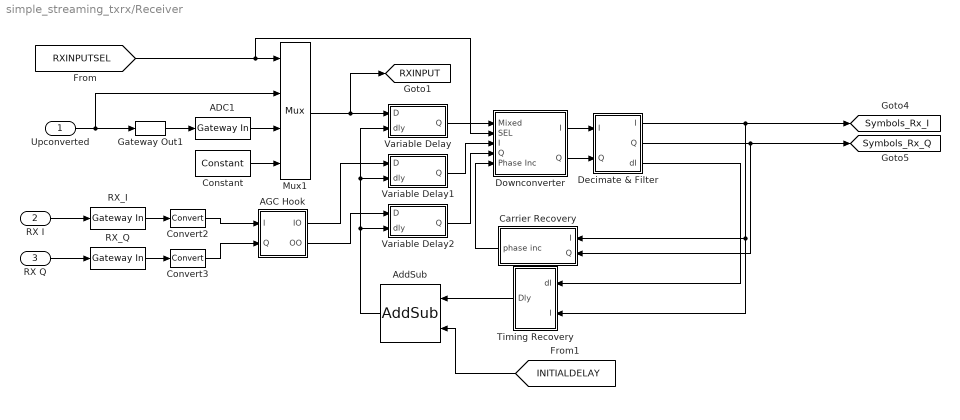
== system simple_streaming_txrx/Receiver ==
  Upconverted : Inport
  RX I : Inport  Port=2
  RX Q : Inport  Port=3
  ADC1 : xbsIndex_r4/Gateway In  arith_type="Signed  (2's comp)"  n_bits=14  bin_pt=13  quantization=Truncate  overflow=Wrap  period=1/8  dbl_ovrd=off  timing_constraint=None  locs_specified=off  LOCs={}  block_type=gatewayin
      settings: infoedit="Gateway in block.  Converts inputs of type Simulink integer, double and fixed point to  Xilinx fixed point type.<P><P>Hardware notes:  In hardware these blocks become top level input ports."  xl_area=[0 0 0 0 14 0 0]  block_version=10.1
  AGC Hook : Subsystem
  AddSub : xbsIndex_r4/AddSub  Orientation=left  mode=Addition  use_carryin=off  use_carryout=off  en=off  latency=0  precision=User Defined  arith_type=Unsigned  n_bits=3  bin_pt=0  quantization=Truncate  overflow=Wrap  dbl_ovrd=off  use_behavioral_HDL=off  pipelined=off  use_rpm=on  block_type=addsub
      settings: xl_area=[2 0 0 3 0 0 0]  block_version=10.1
  Carrier Recovery : Subsystem  Orientation=left
  Constant : xbsIndex_r4/Constant  arith_type=Signed (2's comp)  const=0  n_bits=14  bin_pt=13  explicit_period=off  period=1  equ=P=C  opselect=C  inp2=PCIN>>17  opr=+  inp1=P  carry=CIN  dbl_ovrd=off  block_type=constant
      settings: block_version=10.1
  Convert2 : xbsIndex_r4/Convert  arith_type="Signed  (2's comp)"  n_bits=14  bin_pt=13  quantization=Truncate  overflow=Wrap  latency=0  dbl_ovrd=off  pipeline=off  block_type=convert
      settings: xl_area=[0 0 0 0 0 0 0]  block_version=10.1
  Convert3 : xbsIndex_r4/Convert  arith_type="Signed  (2's comp)"  n_bits=14  bin_pt=13  quantization=Truncate  overflow=Wrap  latency=0  dbl_ovrd=off  pipeline=off  block_type=convert
      settings: xl_area=[0 0 0 0 0 0 0]  block_version=10.1
  Decimate & Filter : Subsystem
  Downconverter : Subsystem
  Gateway Out1 : xbsIndex_r4/Gateway Out  hdl_port=off  timing_constraint=None  locs_specified=off  LOCs={}  block_type=gatewayout
      settings: infoedit="Gateway out block.  Converts Xilinx fixed point inputs into ouputs of type Simulink integer, double, or fixed point.<P><P>Hardware notes:  In hardware these blocks become top level output ports or are discarded, depending on how they are configured."  xl_area=[0 0 0 0 0 0 0]  block_version=10.1
  Mux1 : xbsIndex_r4/Mux  inputs=3  en=off  latency=1  precision=Full  arith_type="Signed  (2's comp)"  n_bits=8  bin_pt=2  quantization=Truncate  overflow=Wrap  dbl_ovrd=off  block_type=mux
      settings: xl_area=[14 14 0 28 0 0 0]  block_version=10.1
  RX_I : xbsIndex_r4/Gateway In  arith_type="Signed  (2's comp)"  n_bits=14  bin_pt=13  quantization=Truncate  overflow=Saturate  period=1/8  dbl_ovrd=off  timing_constraint=None  locs_specified=off  LOCs={}  block_type=gatewayin
      settings: infoedit="Gateway in block.  Converts inputs of type Simulink integer, double and fixed point to  Xilinx fixed point type.<P><P>Hardware notes:  In hardware these blocks become top level input ports."  xl_area=[0 0 0 0 14 0 0]  block_version=10.1
  RX_Q : xbsIndex_r4/Gateway In  arith_type="Signed  (2's comp)"  n_bits=14  bin_pt=13  quantization=Truncate  overflow=Saturate  period=1/8  dbl_ovrd=off  timing_constraint=None  locs_specified=off  LOCs={}  block_type=gatewayin
      settings: infoedit="Gateway in block.  Converts inputs of type Simulink integer, double and fixed point to  Xilinx fixed point type.<P><P>Hardware notes:  In hardware these blocks become top level input ports."  xl_area=[0 0 0 0 14 0 0]  block_version=10.1
  Timing Recovery : Subsystem  Orientation=left
  Variable Delay : Subsystem
  Variable Delay1 : Subsystem
  Variable Delay2 : Subsystem
  tag scope: RXINPUT=global, Symbols_Rx_I=global, Symbols_Rx_Q=global
  wires:
  Upconverted/1 -> Mux1/2, Gateway Out1/1
  Downconverter/1(" I") -> Decimate & Filter/1(I)
  Downconverter/2(" Q") -> Decimate & Filter/2(Q)
  Carrier Recovery/1(" phase inc") -> Downconverter/5(Phase Inc)
  Decimate & Filter/3(" dI") -> Timing Recovery/1(dI)
  [RXINPUTSEL] -> Mux1/1, Downconverter/2(SEL)
  Mux1/1 -> Variable Delay/1(D), [RXINPUT]
  ADC1/1 -> Mux1/3
  Gateway Out1/1 -> ADC1/1
  Timing Recovery/1(Dly) -> AddSub/1
  AddSub/1 -> Variable Delay/2(dly), Variable Delay1/2(dly), Variable Delay2/2(dly)
  [INITIALDELAY] -> AddSub/2
  Variable Delay/1(Q) -> Downconverter/1(Mixed)
  RX I/1 -> RX_I/1
  RX Q/1 -> RX_Q/1
  Constant/1 -> Mux1/4
  RX_I/1 -> Convert2/1
  RX_Q/1 -> Convert3/1
  Variable Delay1/1(Q) -> Downconverter/3(I)
  Variable Delay2/1(Q) -> Downconverter/4(Q)
  Decimate & Filter/1(" I") -> [Symbols_Rx_I], Carrier Recovery/1(I), Timing Recovery/2(I)
  Decimate & Filter/2(" Q") -> [Symbols_Rx_Q], Carrier Recovery/2(Q)
  Convert2/1 -> AGC Hook/1(I)
  Convert3/1 -> AGC Hook/2(Q)
  AGC Hook/1(IO) -> Variable Delay1/1(D)
  AGC Hook/2(OO) -> Variable Delay2/1(D)
